simulink model "pid_example"  (R2023a)
settings: Solver=VariableStepAuto  StartTime=0.0  StopTime=10.0  RelTol=1e-3
undefined symbols (not defined in the file or in its folder): Kp, Td, Ti
settings Model: Creator=pinki  LastModifiedBy=pinki

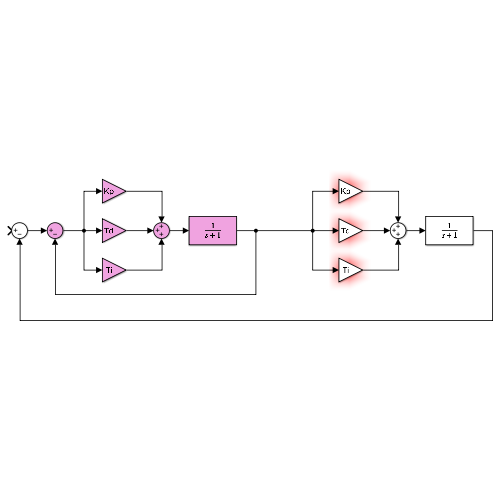
[thumbnail: Simulink's stored preview of the top-level diagram]
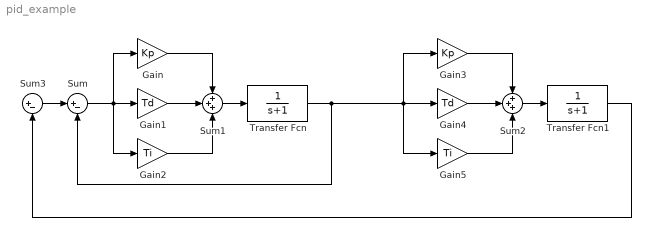
== system pid_example ==
  Gain : Gain  Gain=Kp
  Gain1 : Gain  Gain=Td
  Gain2 : Gain  Gain=Ti
  Gain3 : Gain  Gain=Kp
  Gain4 : Gain  Gain=Td
  Gain5 : Gain  Gain=Ti
  Sum : Sum  Inputs=|+-
  Sum1 : Sum  Inputs=+++
  Sum2 : Sum  Inputs=+++
  Sum3 : Sum  Inputs=|+-
  Transfer Fcn : TransferFcn  Denominator=[1 1]
  Transfer Fcn1 : TransferFcn  Denominator=[1 1]
  wires:
  Sum/1 -> Gain2/1, Gain/1, Gain1/1
  Gain/1 -> Sum1/1
  Gain1/1 -> Sum1/2
  Gain2/1 -> Sum1/3
  Sum1/1 -> Transfer Fcn/1
  Transfer Fcn/1 -> Gain5/1, Gain4/1, Gain3/1, Sum/2
  Gain3/1 -> Sum2/1
  Sum2/1 -> Transfer Fcn1/1
  Gain5/1 -> Sum2/3
  Gain4/1 -> Sum2/2
  Sum3/1 -> Sum/1
  Transfer Fcn1/1 -> Sum3/2
